simulink model "functionSP"  (R2020b)
settings: Solver=FixedStepAuto  StartTime=0.0  StopTime=20  RelTol=1e-3
settings Model: Creator=Robert  LastModifiedBy=Robert

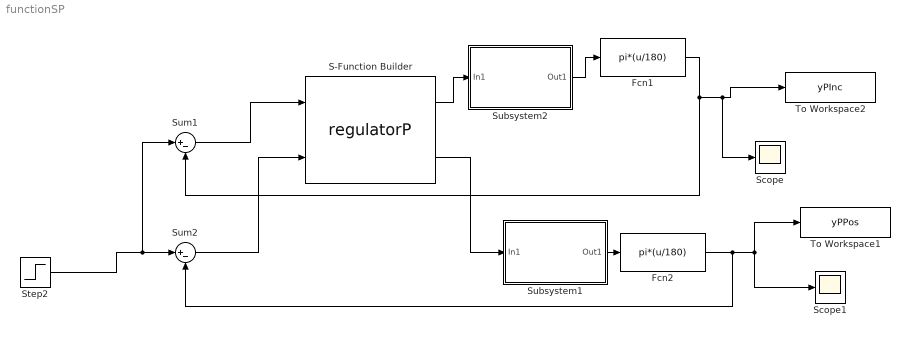
== system functionSP ==
  Fcn1 : Fcn  Expr=pi*(u/180)
  Fcn2 : Fcn  Expr=pi*(u/180)
  S-Function Builder : S-Function  InitFcn=try, set_param(gcb,'FunctionName','regulatorP'), end  FunctionName=regulatorP  Parameters=1.1437,5.5780,1.3945,0.01  SFunctionModules=regulatorP_wrapper  SFunctionDeploymentMode=off  EnableBusSupport=off  mask(S-Function Builder){}
      mask help: Simulink:masks:SFunctionBuilder_MD
      mask init:
      | val = [[.9  0.75 0.75 1 1 .9 .9 1]',[1 1 0.75 0.75 .9 .9 1 .9]'];try , sys = get_param(gcb,'SfunBuilderFcnName');if isempty(sys), sys = get_param(gcb,'FunctionName'); end,catch, sys = get_param(gcb,'FunctionName'); end
      settings: CopyFcn=set_param(gcbh,'LinkStatus','none')  PreSaveFcn=try, set_param(gcb,'FunctionName','regulatorP'), end  OpenFcn=sfunctionwizard(gcbh)
      mask Display: plot(val(:,1),val(:,2)),disp(sys),port_label('input',1,'eInc'),port_label('input',2,'ePos'),port_label('output',1,'yInc'),port_label('output',2,'yPos')
  Scope : Scope
  Scope1 : Scope
  Step2 : Step  Time=0  After=u  SampleTime=0
  Subsystem1 : Subsystem
  Subsystem2 : Subsystem
  Sum1 : Sum  Inputs=|+-
  Sum2 : Sum  Inputs=|+-
  To Workspace1 : ToWorkspace  VariableName=yPPos  SampleTime=-1
      settings: Save2DSignal=2-D array (concatenate along first dimension)
  To Workspace2 : ToWorkspace  VariableName=yPInc  SampleTime=-1
      settings: Save2DSignal=2-D array (concatenate along first dimension)
  wires:
  Step2/1 -> Sum1/1, Sum2/1
  Sum2/1 -> S-Function Builder/2
  Fcn2/1 -> Sum2/2, Scope1/1, To Workspace1/1
  Subsystem1/1(Out1) -> Fcn2/1
  Fcn1/1 -> Scope/1, To Workspace2/1, Sum1/2
  S-Function Builder/2 -> Subsystem1/1(In1)
  Sum1/1 -> S-Function Builder/1
  Subsystem2/1(Out1) -> Fcn1/1
  S-Function Builder/1 -> Subsystem2/1(In1)

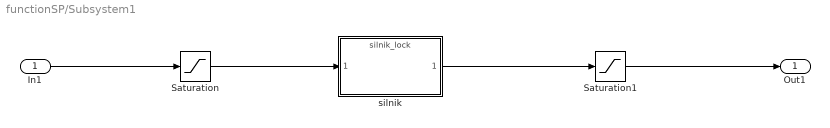
== system functionSP/Subsystem1 ==
  In1 : Inport
  Saturation : Saturate  UpperLimit=2  LowerLimit=-2
  Saturation1 : Saturate  UpperLimit=180  LowerLimit=-180
  silnik : ModelReference  ModelNameDialog=silnik_lock.slxp  ModelReferenceVersion=1.38  CopyOfModelProtected=on
  Out1 : Outport
  wires:
  Saturation/1 -> silnik/1
  In1/1 -> Saturation/1
  silnik/1 -> Saturation1/1
  Saturation1/1 -> Out1/1

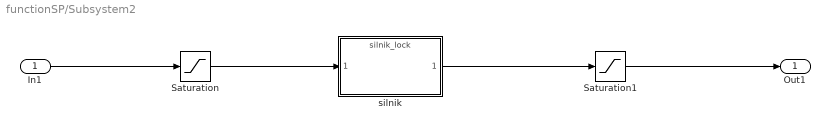
== system functionSP/Subsystem2 ==
  In1 : Inport
  Saturation : Saturate  UpperLimit=2  LowerLimit=-2
  Saturation1 : Saturate  UpperLimit=180  LowerLimit=-180
  silnik : ModelReference  ModelNameDialog=silnik_lock.slxp  ModelReferenceVersion=1.38  CopyOfModelProtected=on
  Out1 : Outport
  wires:
  Saturation/1 -> silnik/1
  In1/1 -> Saturation/1
  silnik/1 -> Saturation1/1
  Saturation1/1 -> Out1/1
